simulink model "IEEE_three_phase_14Bus_test_system_with_harmonics"  (R2016a)
settings: Solver=ode15s  StartTime=0  StopTime=6/60  RelTol=1e-6
libraries: powerlib x127
(part 2 of 2)

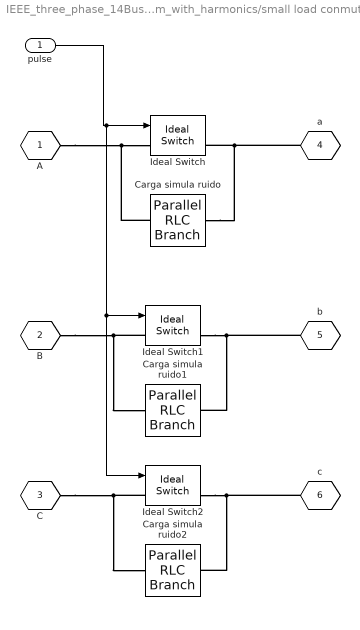
== system IEEE_three_phase_14Bus_test_system_with_harmonics/small load conmuted9 ==
  pulse : Inport
  Carga simula ruido : powerlib/Elements/Parallel RLC Branch  LConnTagsString=a  RConnTagsString=__new0  BranchType=RL  Resistance=2  Inductance=1e-2  SetiL0=off  InitialCurrent=0  Capacitance=0  Setx0=off  InitialVoltage=0  Measurements=None
  Carga simula ruido1 : powerlib/Elements/Parallel RLC Branch  LConnTagsString=a  RConnTagsString=__new0  BranchType=RL  Resistance=2  Inductance=1e-2  SetiL0=off  InitialCurrent=0  Capacitance=0  Setx0=off  InitialVoltage=0  Measurements=None
  Carga simula ruido2 : powerlib/Elements/Parallel RLC Branch  LConnTagsString=a  RConnTagsString=__new0  BranchType=RL  Resistance=2  Inductance=1e-2  SetiL0=off  InitialCurrent=0  Capacitance=0  Setx0=off  InitialVoltage=0  Measurements=None
  Ideal Switch : powerlib/Power Electronics/Ideal Switch  Ron=0.001  Lon=0  IC=0  Rs=1e5  Cs=inf  Measurements=on
  Ideal Switch1 : powerlib/Power Electronics/Ideal Switch  Ron=0.001  Lon=0  IC=0  Rs=1e5  Cs=inf  Measurements=on
  Ideal Switch2 : powerlib/Power Electronics/Ideal Switch  Ron=0.001  Lon=0  IC=0  Rs=1e5  Cs=inf  Measurements=on
  A : PMIOPort  Tag=PMCPort  Port=1  Side=Left
  B : PMIOPort  Tag=PMCPort  Port=2  Side=Left
  C : PMIOPort  Tag=PMCPort  Port=3  Side=Left
  a : PMIOPort  Tag=PMCPort  Port=4  Side=Right
  b : PMIOPort  Tag=PMCPort  Port=5  Side=Right
  c : PMIOPort  Tag=PMCPort  Port=6  Side=Right
  wires:
  pulse/1 -> Ideal Switch2/1, Ideal Switch1/1, Ideal Switch/1
  connections:
  A/RConn1 -- Ideal Switch/LConn1 -- Carga simula ruido/RConn1
  C/RConn1 -- Carga simula ruido2/RConn1 -- Ideal Switch2/LConn1
  B/RConn1 -- Carga simula ruido1/RConn1 -- Ideal Switch1/LConn1
  b/RConn1 -- Carga simula ruido1/LConn1 -- Ideal Switch1/RConn1
  c/RConn1 -- Carga simula ruido2/LConn1 -- Ideal Switch2/RConn1
  a/RConn1 -- Ideal Switch/RConn1 -- Carga simula ruido/LConn1
